simulink model "SwitchingPattern_NPC_CarrierBased"  (R2023b)
settings: Solver=ode45  StartTime=0.0  StopTime=0.2  RelTol=1e-3
InitFcn:
  | %% Switching pattern Variables
  | 
  | % Grid Frequency
  | F_grid = 50 ; % [Hz]
  | Sine_amplide_scaler = 1.1;
  | third_Harmonic_scaler = 1/6 ; % normal 0.15-0.2
  | 
  | % [V] : Voltage DC-Link
  | V_dc = 5000 ;
  | 
  | % Condensator (and Resistor) holding the neutralpoint of the npc topology
  | C_NPC = 3300e-3;
  | R_NPC = 1E-3 ;
  | 
  | % Switching Frequency
  | F_sw = 1500 ; % [Hz]
  | T_sw = 1/F_sw ;
  | 
  | % LC Filter Inductor
  | L_Filter_NPC = 5e-3;   %5e-3 ;
  | C_Filter_NPC = 0;      %3e-6 ;
  | R_Filter_NPC = inf;    %1E-3 ;
  | 
  | % Sine time steps
  | sample_time = 10E-6;%1E-6 ; % should match the discrete solver time steps
  | 
  | % Dead Time Insertion for IGBTs
  | dead_time = 3E-6 ; % normal 2-4us
StopFcn:
  | Vout_scope = out.Vout_ScopeData ;
libraries: spsOnDelayLib x12, spsIGBTDiodeLib x12, spsSeriesRLCBranchLib x9, spsDiodeLib x6, spsVoltageMeasurementLib x4, spsCurrentMeasurementLib x3, simulink x2, spsDCVoltageSourceLib x1, spsThreePhaseSeriesRLCBranchLib x1, spsThreePhaseVIMeasurementLib x1, spspowerguiLib x1
settings Model: Creator=leons  LastModifiedBy=leons

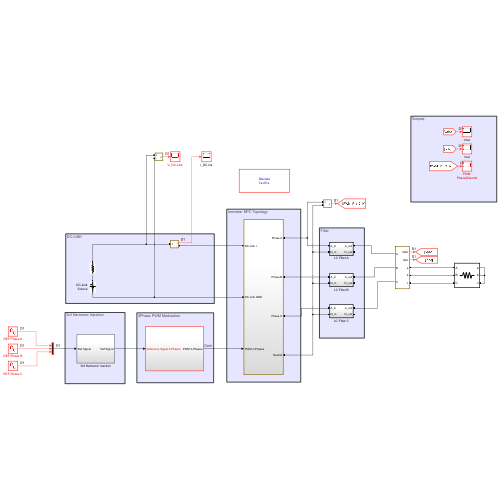
[thumbnail: Simulink's stored preview of the top-level diagram]
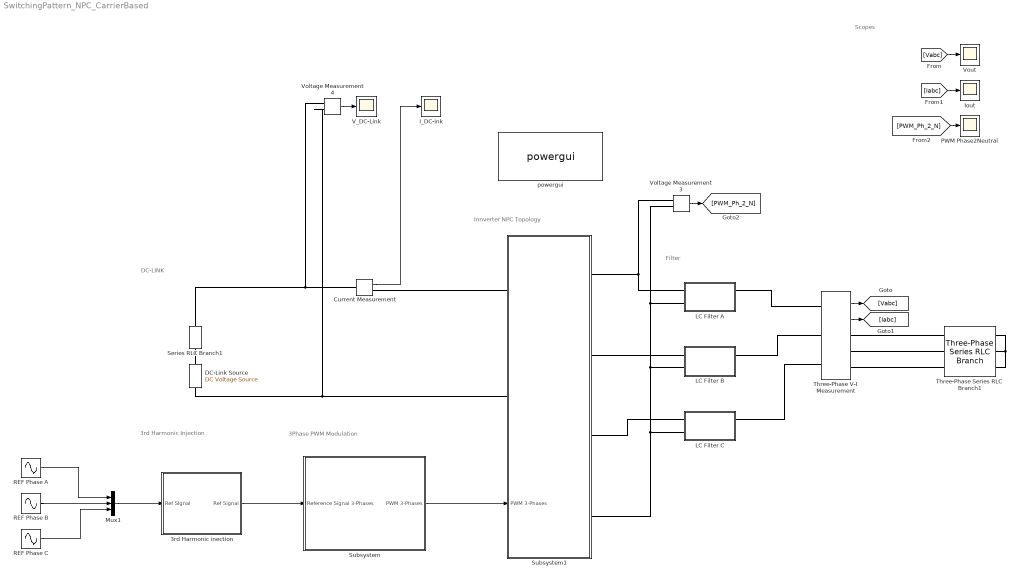
== system SwitchingPattern_NPC_CarrierBased ==
  note: Scopes
  note: Innverter NPC Topology
  note: DC-LINK
  note: 3rd Harmonic Injection
  note: Filter
  note: 3Phase PWM Modulation
  3rd Harmonic inection : Subsystem
  Current Measurement : spsCurrentMeasurementLib/Current Measurement  PhasorSimulation=off  OutputType=Complex  PSBequivalent=0
  DC-Link Source : spsDCVoltageSourceLib/DC Voltage Source  Amplitude=V_dc  Measurements=None
  I_DC-ink : Scope
  Iout : Scope
  LC Filter A : Subsystem
  LC Filter B : Subsystem
  LC Filter C : Subsystem
  Mux1 : Mux  Inputs=3
  PWM Phase2Neutral : Scope
  REF Phase A : Sin  Amplitude=0.5*Sine_amplide_scaler  Bias=0.5  Frequency=2*pi*F_grid  SampleTime=sample_time
  REF Phase B : Sin  Amplitude=0.5*Sine_amplide_scaler  Bias=0.5  Frequency=2*pi*F_grid  Phase=2*pi/3  SampleTime=sample_time
  REF Phase C : Sin  Amplitude=0.5*Sine_amplide_scaler  Bias=0.5  Frequency=2*pi*F_grid  Phase=4*pi/3  SampleTime=sample_time
  Series RLC Branch1 : spsSeriesRLCBranchLib/Series RLC Branch  LConnTagsString=__new0  RConnTagsString=__new0  BranchType=R  Resistance=R_NPC  Inductance=1e-3  SetiL0=off  InitialCurrent=0  Capacitance=470e-6  Setx0=off  InitialVoltage=0  Measurements=None
  Subsystem : Subsystem
  Subsystem1 : Subsystem
      settings: PortSchema="{\"entries\":[{\"content\":{\"sides\":[{\"content\":{\"connectorIds\":[\"LConn1\",\"LConn2\",\"In1\"]},\"type\":\"ConnectorPlacement.EquallySpacedRectSide\",\"uuid\":\"3d46b57d-d8b7-49b7-aaf6-608df73eb91e\"},{\"content\":{\"connectorIds\":[\"RConn1\",\"RConn2\",\"RConn3\",\"RConn4\"],\"side\":\"RIGHT\"},\"type\":\"ConnectorPlacement.EquallySpacedRectSide\",\"uuid\":\"1122e1de-704f-4457-b1d2-7bb2957c0af7\"},{\"content\":{\"side\":\"TOP\"},\"type\":\"ConnectorPlacement.EquallySpacedRectSide\",\"uuid\":\"4106d887-06ba-41de-a617-0ceeae9667fe\"}]},\"type\":\"ConnectorPlacement.EquallySpacedConnector\",\"uuid\":\"eb31d605-2a54-43c7-b39a-3ef79e5e21b2\"}],\"packageUris\":[\"http://schema.mathworks.com/mf0/Connector/R2020b\"],\"version\":\"1.0\"}"
  Three-Phase Series RLC Branch1 : spsThreePhaseSeriesRLCBranchLib/Three-Phase Series RLC Branch  LConnTagsString=A|B|C  RConnTagsString=A|B|C  BranchType=R  Resistance=1  Inductance=1e-3  Capacitance=1e-6  Measurements=None
  Three-Phase V-I Measurement : spsThreePhaseVIMeasurementLib/Three-Phase V-I Measurement  VoltageMeasurement=phase-to-phase  SetLabelV=off  LabelV=Vabc  Vpu=off  VpuLL=off  CurrentMeasurement=yes  SetLabelI=off  LabelI=Iabc  Ipu=off  Pbase=100e6  Vbase=500e3  OutputType=Complex  PhasorSimulation=off  PSBequivalent=0
  V_DC-Link : Scope
  Voltage Measurement3 : spsVoltageMeasurementLib/Voltage Measurement  PhasorSimulation=off  OutputType=Complex  PSBequivalent=0
  Voltage Measurement4 : spsVoltageMeasurementLib/Voltage Measurement  PhasorSimulation=off  OutputType=Complex  PSBequivalent=0
  Vout : Scope
  powergui : spspowerguiLib/powergui  Priority=1  SimulationMode=Discrete  SampleTime=sample_time  frequency=60  Iterations=50  frequencyindice=0  Pbase=100e6  ErrMax=1e-4  UnitsV=kV  UnitsW=MW  buscounter=0  FunctionMessages=off  echomessages=off  EnableUseOfTLC=off  CurrentSourceSwitches=off  DisableSnubberDevices=off  DisableRonSwitches=off  DisableVfSwitches=off  DisplayEquations=off  AutomaticDiscreteSolvers=off  SolverType=Tustin/Backward Euler (TBE)  Interpol=off  ExternalGateDelay=off  methode=off  Ts=100  x0status=blocks  SPID=on  SwTol=0  HookPort=off  NonlinearTolerance=1e-4  nMaxIteration=100  ContinueOnMaxIteration=off  RestoreLinks=warning  ResistiveCurrentMeasurement=off  Frange=[0:2:500]  Ylog=off  Xlog=on  ShowGrid=off  save=off  variable=ZData  structure=0  ZoomFFT=off  StartTime=0.0  cycles=1  DisplayStyle=1  fundamental=60  FreqAxis=off  MaxFrequency=1000  frequencyindicesteady=1  RmsSteady=1  display=off
  wires:
  Voltage Measurement3/1 -> [PWM_Ph_2_N]
  Voltage Measurement4/1 -> V_DC-Link/1
  Current Measurement/1 -> I_DC-ink/1
  Subsystem/1(PWM 3-Phases) -> Subsystem1/1(PWM 3-Phases)
  REF Phase A/1 -> Mux1/1
  REF Phase B/1 -> Mux1/2
  REF Phase C/1 -> Mux1/3
  Three-Phase V-I Measurement/1 -> [Vabc]
  Three-Phase V-I Measurement/2 -> [Iabc]
  [Vabc] -> Vout/1
  [Iabc] -> Iout/1
  [PWM_Ph_2_N] -> PWM Phase2Neutral/1
  Mux1/1 -> 3rd Harmonic inection/1(Ref SIgnal)
  3rd Harmonic inection/1(Ref Signal) -> Subsystem/1(Reference Signal 3-Phases)
  connections:
  Voltage Measurement3/LConn1 -- Subsystem1/RConn1 -- LC Filter A/LConn1
  LC Filter A/RConn1 -- Three-Phase V-I Measurement/LConn1
  LC Filter B/RConn1 -- Three-Phase V-I Measurement/LConn2
  LC Filter C/RConn1 -- Three-Phase V-I Measurement/LConn3
  Three-Phase Series RLC Branch1/LConn1 -- Three-Phase V-I Measurement/RConn1
  Three-Phase V-I Measurement/RConn2 -- Three-Phase Series RLC Branch1/LConn2
  Three-Phase V-I Measurement/RConn3 -- Three-Phase Series RLC Branch1/LConn3
  Three-Phase Series RLC Branch1/RConn1 -- Three-Phase Series RLC Branch1/RConn3 -- Three-Phase Series RLC Branch1/RConn2
  Series RLC Branch1/LConn1 -- Voltage Measurement4/LConn1 -- Current Measurement/LConn1
  DC-Link Source/RConn1 -- Series RLC Branch1/RConn1
  Voltage Measurement4/LConn2 -- DC-Link Source/LConn1 -- Subsystem1/LConn2
  Subsystem1/LConn1 -- Current Measurement/RConn1
  Subsystem1/RConn2 -- LC Filter B/LConn1
  Subsystem1/RConn3 -- LC Filter C/LConn1
  LC Filter A/LConn2 -- Voltage Measurement3/LConn2 -- Subsystem1/RConn4 -- LC Filter C/LConn2 -- LC Filter B/LConn2

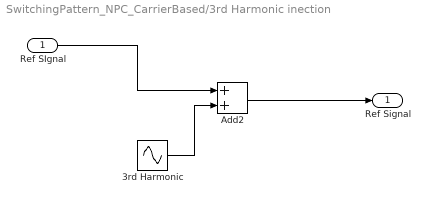
== system SwitchingPattern_NPC_CarrierBased/3rd Harmonic inection ==
  Ref SIgnal : Inport
  3rd Harmonic : Sin  Amplitude=0.5*Sine_amplide_scaler*third_Harmonic_scaler  Frequency=3*2*pi*F_grid  SampleTime=sample_time
  Add2 : Sum
  Ref Signal : Outport
  wires:
  3rd Harmonic/1 -> Add2/2
  Add2/1 -> Ref Signal/1
  Ref SIgnal/1 -> Add2/1

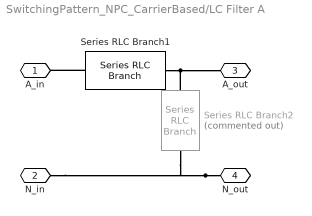
== system SwitchingPattern_NPC_CarrierBased/LC Filter A ==
  Series RLC Branch1 : spsSeriesRLCBranchLib/Series RLC Branch  LConnTagsString=__new0  RConnTagsString=__new0  BranchType=L  Resistance=1  Inductance=L_Filter_NPC  SetiL0=off  InitialCurrent=0  Capacitance=1e-6  Setx0=off  InitialVoltage=0  Measurements=None
  Series RLC Branch2 : spsSeriesRLCBranchLib/Series RLC Branch  Commented=on  LConnTagsString=__new0  RConnTagsString=__new0  BranchType=RC  Resistance=R_Filter_NPC  Inductance=1e-3  SetiL0=off  InitialCurrent=0  Capacitance=C_Filter_NPC  Setx0=off  InitialVoltage=V_dc/2  Measurements=None
  A_in : PMIOPort  Side=Left
  N_in : PMIOPort  Port=2  Side=Left
  A_out : PMIOPort  Port=3  Side=Right
  N_out : PMIOPort  Port=4  Side=Right
  connections:
  Series RLC Branch1/RConn1 -- Series RLC Branch2/LConn1 -- A_out/RConn1
  N_out/RConn1 -- Series RLC Branch2/RConn1 -- N_in/RConn1
  Series RLC Branch1/LConn1 -- A_in/RConn1

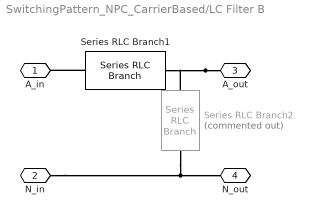
== system SwitchingPattern_NPC_CarrierBased/LC Filter B ==
  Series RLC Branch1 : spsSeriesRLCBranchLib/Series RLC Branch  LConnTagsString=__new0  RConnTagsString=__new0  BranchType=L  Resistance=1  Inductance=L_Filter_NPC  SetiL0=off  InitialCurrent=0  Capacitance=1e-6  Setx0=off  InitialVoltage=0  Measurements=None
  Series RLC Branch2 : spsSeriesRLCBranchLib/Series RLC Branch  Commented=on  LConnTagsString=__new0  RConnTagsString=__new0  BranchType=RC  Resistance=R_Filter_NPC  Inductance=1e-3  SetiL0=off  InitialCurrent=0  Capacitance=C_Filter_NPC  Setx0=off  InitialVoltage=V_dc/2  Measurements=None
  A_in : PMIOPort  Side=Left
  N_in : PMIOPort  Port=2  Side=Left
  A_out : PMIOPort  Port=3  Side=Right
  N_out : PMIOPort  Port=4  Side=Right
  connections:
  Series RLC Branch1/LConn1 -- A_in/RConn1
  N_in/RConn1 -- Series RLC Branch2/RConn1 -- N_out/RConn1
  A_out/RConn1 -- Series RLC Branch2/LConn1 -- Series RLC Branch1/RConn1

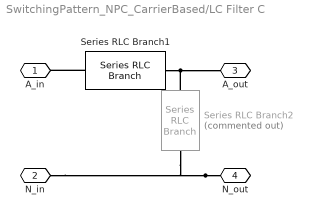
== system SwitchingPattern_NPC_CarrierBased/LC Filter C ==
  Series RLC Branch1 : spsSeriesRLCBranchLib/Series RLC Branch  LConnTagsString=__new0  RConnTagsString=__new0  BranchType=L  Resistance=1  Inductance=L_Filter_NPC  SetiL0=off  InitialCurrent=0  Capacitance=1e-6  Setx0=off  InitialVoltage=0  Measurements=None
  Series RLC Branch2 : spsSeriesRLCBranchLib/Series RLC Branch  Commented=on  LConnTagsString=__new0  RConnTagsString=__new0  BranchType=RC  Resistance=R_Filter_NPC  Inductance=1e-3  SetiL0=off  InitialCurrent=0  Capacitance=C_Filter_NPC  Setx0=off  InitialVoltage=V_dc/2  Measurements=None
  A_in : PMIOPort  Side=Left
  N_in : PMIOPort  Port=2  Side=Left
  A_out : PMIOPort  Port=3  Side=Right
  N_out : PMIOPort  Port=4  Side=Right
  connections:
  Series RLC Branch1/RConn1 -- Series RLC Branch2/LConn1 -- A_out/RConn1
  N_out/RConn1 -- Series RLC Branch2/RConn1 -- N_in/RConn1
  Series RLC Branch1/LConn1 -- A_in/RConn1

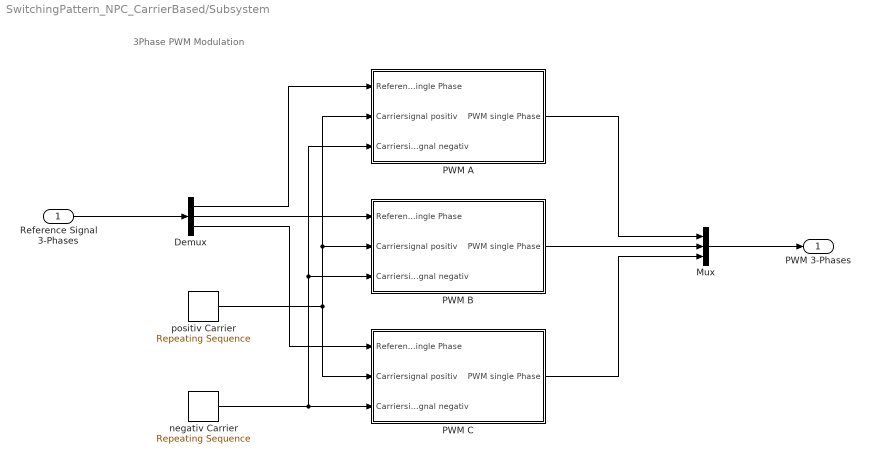
== system SwitchingPattern_NPC_CarrierBased/Subsystem ==
  note: 3Phase PWM Modulation
  Reference Signal 3-Phases : Inport
  Demux : Demux  Outputs=3
  Mux : Mux  Inputs=3
  "PWM A " : Subsystem
  PWM B : Subsystem
  PWM C : Subsystem
  negativ Carrier : simulink/Sources/Repeating Sequence  rep_seq_t=[0 0.5 1]*T_sw  rep_seq_y=[0.5 0 0.5]
  positiv Carrier : simulink/Sources/Repeating Sequence  rep_seq_t=[0 0.5 1]*T_sw  rep_seq_y=[0.5 1 0.5]
  PWM 3-Phases : Outport
  wires:
  positiv Carrier/1 -> PWM C/2(Carriersignal positiv), PWM B/2(Carriersignal positiv), "PWM A "/2(Carriersignal positiv)
  PWM C/1(PWM single Phase) -> Mux/3
  negativ Carrier/1 -> PWM C/3(Carriersignal negativ), PWM B/3(Carriersignal negativ), "PWM A "/3(Carriersignal negativ)
  Demux/2 -> PWM B/1(Reference Signal single Phase)
  "PWM A "/1(PWM single Phase) -> Mux/1
  Mux/1 -> PWM 3-Phases/1
  Reference Signal 3-Phases/1 -> Demux/1
  Demux/1 -> "PWM A "/1(Reference Signal single Phase)
  Demux/3 -> PWM C/1(Reference Signal single Phase)
  PWM B/1(PWM single Phase) -> Mux/2

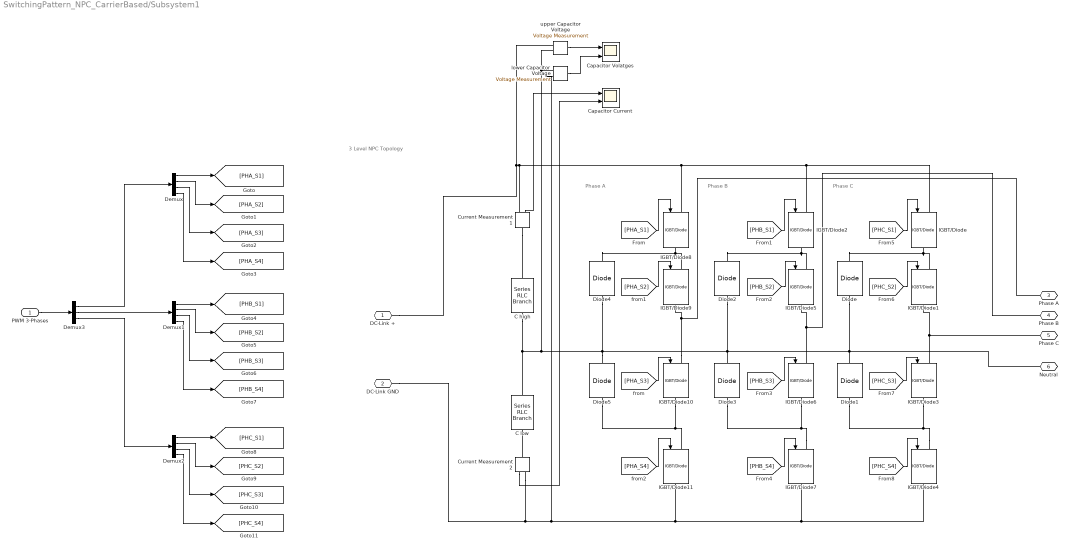
== system SwitchingPattern_NPC_CarrierBased/Subsystem1 ==
  note: 3 Level NPC Topology
  note: Phase C
  note: Phase B
  note: Phase A
  PWM 3-Phases : Inport
  C high : spsSeriesRLCBranchLib/Series RLC Branch  LConnTagsString=__new0  RConnTagsString=__new0  BranchType=C  Resistance=R_NPC  Inductance=1e-3  SetiL0=off  InitialCurrent=0  Capacitance=C_NPC  Setx0=on  InitialVoltage=V_dc/2  Measurements=None
  C low : spsSeriesRLCBranchLib/Series RLC Branch  LConnTagsString=__new0  RConnTagsString=__new0  BranchType=C  Resistance=R_NPC  Inductance=1e-3  SetiL0=off  InitialCurrent=0  Capacitance=C_NPC  Setx0=on  InitialVoltage=V_dc/2  Measurements=None
  Capacitor Current : Scope  NumInputPorts=2
  Capacitor Volatges : Scope  NumInputPorts=2
  Current Measurement1 : spsCurrentMeasurementLib/Current Measurement  PhasorSimulation=off  OutputType=Complex  PSBequivalent=0
  Current Measurement2 : spsCurrentMeasurementLib/Current Measurement  PhasorSimulation=off  OutputType=Complex  PSBequivalent=0
  Demux : Demux
  Demux1 : Demux
  Demux2 : Demux
  Demux3 : Demux  Outputs=3
  Diode{,1..5} (6 alike) : spsDiodeLib/Diode  Ron=0.001  Lon=0  Vf=0.8  IC=0  UseSnubber=0  Rs=500  Cs=250e-9  Measurements=off
  IGBT/Diode{,1..11} (12 alike) : spsIGBTDiodeLib/IGBT//Diode  Ron=1e-3  Rs=1e5  Cs=inf  Measurements=off
  lower Capacitor Voltage : spsVoltageMeasurementLib/Voltage Measurement  PhasorSimulation=off  OutputType=Complex  PSBequivalent=0
  upper Capacitor Voltage : spsVoltageMeasurementLib/Voltage Measurement  PhasorSimulation=off  OutputType=Complex  PSBequivalent=0
  DC-Link + : PMIOPort  Side=Left
  DC-Link GND : PMIOPort  Port=2  Side=Left
  Phase A : PMIOPort  Port=3  Side=Right
  Phase B : PMIOPort  Port=4  Side=Right
  Phase C : PMIOPort  Port=5  Side=Right
  Neutral : PMIOPort  Port=6  Side=Right
  wires:
  [PHC_S2] -> IGBT/Diode1/1
  [PHC_S3] -> IGBT/Diode3/1
  Current Measurement2/1 -> Capacitor Current/2
  [PHB_S4] -> IGBT/Diode7/1
  [PHB_S2] -> IGBT/Diode5/1
  Demux2/2 -> [PHC_S2]
  Demux2/4 -> [PHC_S4]
  [PHC_S1] -> IGBT/Diode/1
  [PHB_S3] -> IGBT/Diode6/1
  Demux/4 -> [PHA_S4]
  Demux/1 -> [PHA_S1]
  Demux/3 -> [PHA_S3]
  [PHA_S1] -> IGBT/Diode8/1
  upper Capacitor Voltage/1 -> Capacitor Volatges/1
  Demux2/3 -> [PHC_S3]
  [PHB_S1] -> IGBT/Diode2/1
  Current Measurement1/1 -> Capacitor Current/1
  Demux1/2 -> [PHB_S2]
  Demux1/3 -> [PHB_S3]
  Demux1/1 -> [PHB_S1]
  [PHA_S4] -> IGBT/Diode11/1
  Demux2/1 -> [PHC_S1]
  Demux1/4 -> [PHB_S4]
  [PHA_S2] -> IGBT/Diode9/1
  lower Capacitor Voltage/1 -> Capacitor Volatges/2
  Demux/2 -> [PHA_S2]
  [PHC_S4] -> IGBT/Diode4/1
  [PHA_S3] -> IGBT/Diode10/1
  PWM 3-Phases/1 -> Demux3/1
  Demux3/1 -> Demux/1
  Demux3/2 -> Demux1/1
  Demux3/3 -> Demux2/1
  connections:
  lower Capacitor Voltage/LConn2 -- DC-Link GND/RConn1 -- Current Measurement2/RConn1 -- IGBT/Diode11/RConn1 -- IGBT/Diode7/RConn1 -- IGBT/Diode4/RConn1
  IGBT/Diode4/LConn1 -- Diode1/LConn1 -- IGBT/Diode3/RConn1
  Diode5/RConn1 -- Diode4/LConn1 -- Neutral/RConn1 -- Diode/LConn1 -- Diode1/RConn1 -- Diode2/LConn1 -- Diode3/RConn1 -- upper Capacitor Voltage/LConn2 -- lower Capacitor Voltage/LConn1 -- C high/RConn1 -- C low/LConn1
  IGBT/Diode10/LConn1 -- Phase A/RConn1 -- IGBT/Diode9/RConn1
  IGBT/Diode10/RConn1 -- IGBT/Diode11/LConn1 -- Diode5/LConn1
  IGBT/Diode/RConn1 -- Diode/RConn1 -- IGBT/Diode1/LConn1
  IGBT/Diode5/RConn1 -- Phase B/RConn1 -- IGBT/Diode6/LConn1
  IGBT/Diode7/LConn1 -- Diode3/LConn1 -- IGBT/Diode6/RConn1
  IGBT/Diode8/LConn1 -- DC-Link +/RConn1 -- upper Capacitor Voltage/LConn1 -- Current Measurement1/RConn1 -- IGBT/Diode2/LConn1 -- IGBT/Diode/LConn1
  Current Measurement1/LConn1 -- C high/LConn1
  IGBT/Diode2/RConn1 -- Diode2/RConn1 -- IGBT/Diode5/LConn1
  IGBT/Diode9/LConn1 -- IGBT/Diode8/RConn1 -- Diode4/RConn1
  IGBT/Diode1/RConn1 -- Phase C/RConn1 -- IGBT/Diode3/LConn1
  Current Measurement2/LConn1 -- C low/RConn1

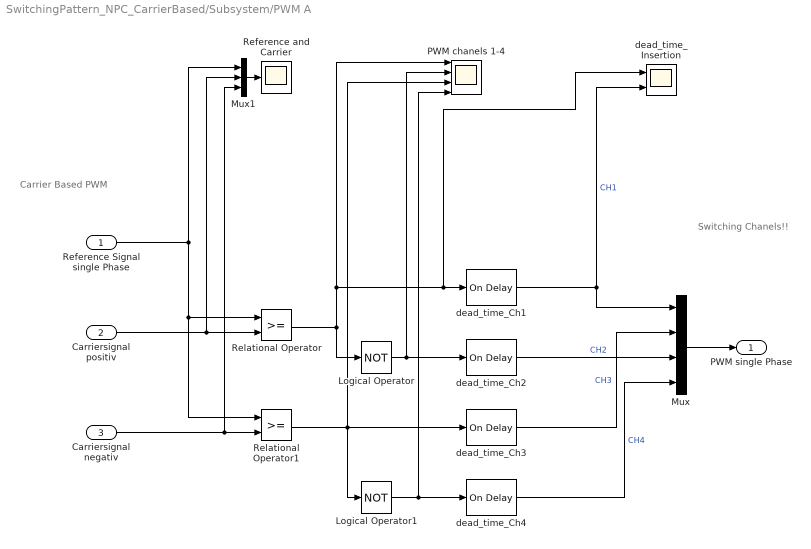
== system SwitchingPattern_NPC_CarrierBased/Subsystem/PWM A  ==
  note: Switching Chanels!!
  note: Carrier Based PWM
  Reference Signal single Phase : Inport
  Carriersignal positiv : Inport  Port=2
  Carriersignal negativ : Inport  Port=3
  Logical Operator : Logic  Operator=NOT  AllPortsSameDT=off  OutDataTypeStr=boolean
  Logical Operator1 : Logic  Operator=NOT  AllPortsSameDT=off  OutDataTypeStr=boolean
  Mux : Mux
  Mux1 : Mux  Inputs=3
  PWM chanels 1-4 : Scope  NumInputPorts=4
  Reference and Carrier : Scope
  Relational Operator : RelationalOperator  OutDataTypeStr=boolean  RndMeth=Simplest  InputSameDT=off
  Relational Operator1 : RelationalOperator  OutDataTypeStr=boolean  RndMeth=Simplest  InputSameDT=off
  dead_time_Ch{1..4} (4 alike) : spsOnDelayLib/On Delay  DelayType=On delay  delay=dead_time  ic=0  Ts=0
  dead_time_Insertion : Scope  NumInputPorts=2
  PWM single Phase : Outport
  wires:
  Relational Operator/1 -> Logical Operator/1, PWM chanels 1-4/1, dead_time_Ch1/1, dead_time_Insertion/1
  Carriersignal negativ/1 -> Mux1/3, Relational Operator1/2
  Carriersignal positiv/1 -> Relational Operator/2, Mux1/2
  dead_time_Ch1/1 -> Mux/1, dead_time_Insertion/2  "CH1"
  Logical Operator/1 -> dead_time_Ch2/1, PWM chanels 1-4/2
  dead_time_Ch2/1 -> Mux/3  "CH2"
  Relational Operator1/1 -> dead_time_Ch3/1, PWM chanels 1-4/3, Logical Operator1/1
  dead_time_Ch3/1 -> Mux/2  "CH3"
  Logical Operator1/1 -> dead_time_Ch4/1, PWM chanels 1-4/4
  dead_time_Ch4/1 -> Mux/4  "CH4"
  Reference Signal single Phase/1 -> Mux1/1, Relational Operator1/1, Relational Operator/1
  Mux/1 -> PWM single Phase/1
  Mux1/1 -> Reference and Carrier/1

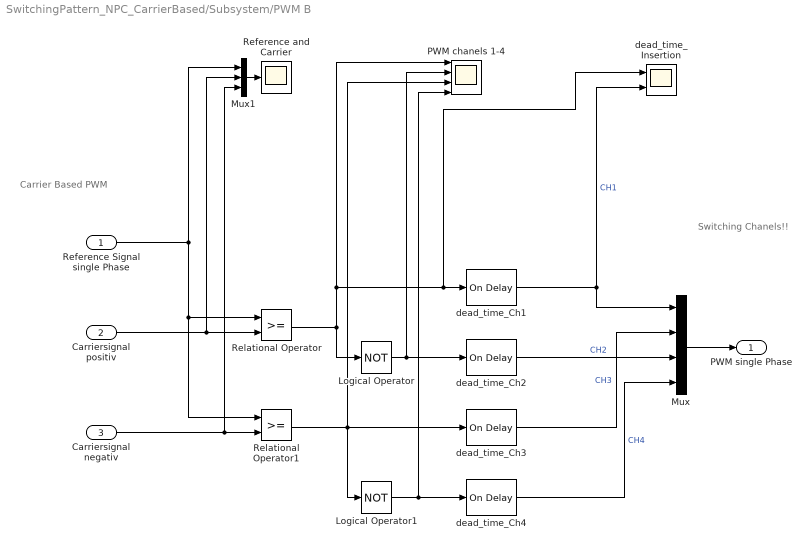
== system SwitchingPattern_NPC_CarrierBased/Subsystem/PWM B ==
  note: Switching Chanels!!
  note: Carrier Based PWM
  Reference Signal single Phase : Inport
  Carriersignal positiv : Inport  Port=2
  Carriersignal negativ : Inport  Port=3
  Logical Operator : Logic  Operator=NOT  AllPortsSameDT=off  OutDataTypeStr=boolean
  Logical Operator1 : Logic  Operator=NOT  AllPortsSameDT=off  OutDataTypeStr=boolean
  Mux : Mux
  Mux1 : Mux  Inputs=3
  PWM chanels 1-4 : Scope  NumInputPorts=4
  Reference and Carrier : Scope
  Relational Operator : RelationalOperator  OutDataTypeStr=boolean  RndMeth=Simplest  InputSameDT=off
  Relational Operator1 : RelationalOperator  OutDataTypeStr=boolean  RndMeth=Simplest  InputSameDT=off
  dead_time_Ch{1..4} (4 alike) : spsOnDelayLib/On Delay  DelayType=On delay  delay=dead_time  ic=0  Ts=0
  dead_time_Insertion : Scope  NumInputPorts=2
  PWM single Phase : Outport
  wires:
  Relational Operator/1 -> Logical Operator/1, PWM chanels 1-4/1, dead_time_Ch1/1, dead_time_Insertion/1
  Carriersignal negativ/1 -> Mux1/3, Relational Operator1/2
  Carriersignal positiv/1 -> Relational Operator/2, Mux1/2
  dead_time_Ch1/1 -> Mux/1, dead_time_Insertion/2  "CH1"
  Logical Operator/1 -> dead_time_Ch2/1, PWM chanels 1-4/2
  dead_time_Ch2/1 -> Mux/3  "CH2"
  Relational Operator1/1 -> dead_time_Ch3/1, PWM chanels 1-4/3, Logical Operator1/1
  dead_time_Ch3/1 -> Mux/2  "CH3"
  Logical Operator1/1 -> dead_time_Ch4/1, PWM chanels 1-4/4
  dead_time_Ch4/1 -> Mux/4  "CH4"
  Reference Signal single Phase/1 -> Mux1/1, Relational Operator1/1, Relational Operator/1
  Mux/1 -> PWM single Phase/1
  Mux1/1 -> Reference and Carrier/1

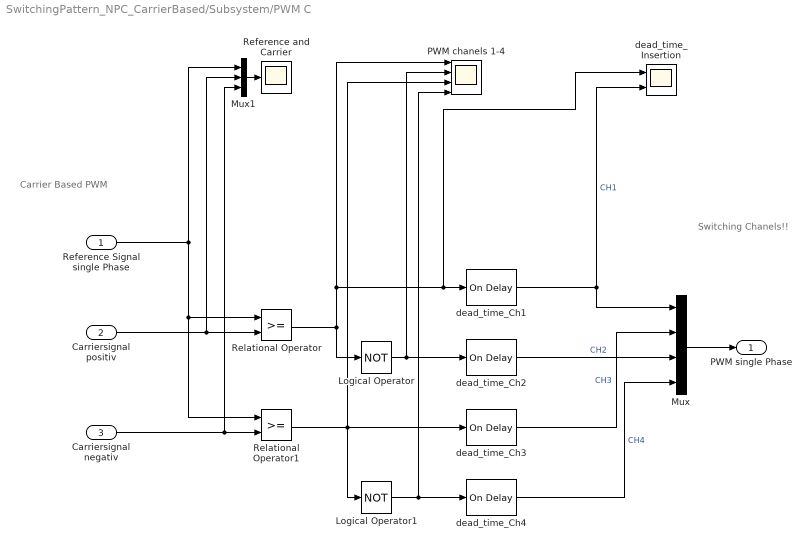
== system SwitchingPattern_NPC_CarrierBased/Subsystem/PWM C ==
  note: Switching Chanels!!
  note: Carrier Based PWM
  Reference Signal single Phase : Inport
  Carriersignal positiv : Inport  Port=2
  Carriersignal negativ : Inport  Port=3
  Logical Operator : Logic  Operator=NOT  AllPortsSameDT=off  OutDataTypeStr=boolean
  Logical Operator1 : Logic  Operator=NOT  AllPortsSameDT=off  OutDataTypeStr=boolean
  Mux : Mux
  Mux1 : Mux  Inputs=3
  PWM chanels 1-4 : Scope  NumInputPorts=4
  Reference and Carrier : Scope
  Relational Operator : RelationalOperator  OutDataTypeStr=boolean  RndMeth=Simplest  InputSameDT=off
  Relational Operator1 : RelationalOperator  OutDataTypeStr=boolean  RndMeth=Simplest  InputSameDT=off
  dead_time_Ch{1..4} (4 alike) : spsOnDelayLib/On Delay  DelayType=On delay  delay=dead_time  ic=0  Ts=0
  dead_time_Insertion : Scope  NumInputPorts=2
  PWM single Phase : Outport
  wires:
  Relational Operator/1 -> Logical Operator/1, PWM chanels 1-4/1, dead_time_Ch1/1, dead_time_Insertion/1
  Carriersignal negativ/1 -> Mux1/3, Relational Operator1/2
  Carriersignal positiv/1 -> Relational Operator/2, Mux1/2
  dead_time_Ch1/1 -> Mux/1, dead_time_Insertion/2  "CH1"
  Logical Operator/1 -> dead_time_Ch2/1, PWM chanels 1-4/2
  dead_time_Ch2/1 -> Mux/3  "CH2"
  Relational Operator1/1 -> dead_time_Ch3/1, PWM chanels 1-4/3, Logical Operator1/1
  dead_time_Ch3/1 -> Mux/2  "CH3"
  Logical Operator1/1 -> dead_time_Ch4/1, PWM chanels 1-4/4
  dead_time_Ch4/1 -> Mux/4  "CH4"
  Reference Signal single Phase/1 -> Mux1/1, Relational Operator1/1, Relational Operator/1
  Mux/1 -> PWM single Phase/1
  Mux1/1 -> Reference and Carrier/1
